simulink model "librarySample"  (R2017b)
settings: Solver=ode3  StartTime=0.0  StopTime=10.0  FixedStep=0.001  RelTol=1e-3
settings Model: Creator=Administrator  LastModifiedBy=Administrator

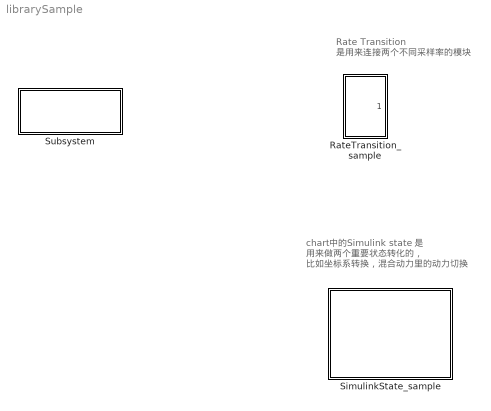
== system librarySample ==
  note: chart中的Simulink state 是
      | 用来做两个重要状态转化的，
      | 比如坐标系转换，混合动力里的动力切换
  note: Rate Transition
      | 是用来连接两个不同采样率的模块
  RateTransition_sample : Subsystem
  SimulinkState_sample : Subsystem
  Subsystem : Subsystem

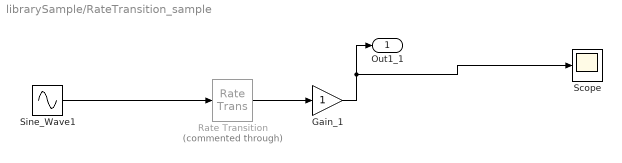
== system librarySample/RateTransition_sample ==
  Gain_1 : Gain
  Rate Transition : RateTransition  Commented=through
  Scope : Scope
  Sine_Wave1 : Sin  SampleTime=0.01
  Out1_1 : Outport  SampleTime=0.1
  wires:
  Sine_Wave1/1 -> Rate Transition/1
  Rate Transition/1 -> Gain_1/1
  Gain_1/1 -> Scope/1, Out1_1/1

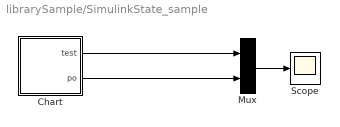
== system librarySample/SimulinkState_sample ==
  Chart : Stateflow chart  TreatAsAtomicUnit=on
  Mux : Mux  Inputs=2
  Scope : Scope
  wires:
  Chart/2(po) -> Mux/2
  Mux/1 -> Scope/1
  Chart/1(test) -> Mux/1

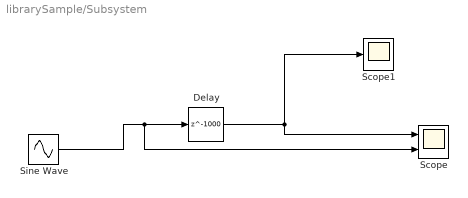
== system librarySample/Subsystem ==
  Delay : Delay  DelayLength=1000
  Scope : Scope  NumInputPorts=2
  Scope1 : Scope
  Sine Wave : Sin  SampleTime=0
  wires:
  Sine Wave/1 -> Scope/2, Delay/1
  Delay/1 -> Scope/1, Scope1/1

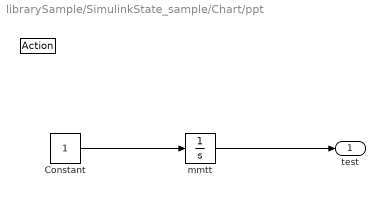
== system librarySample/SimulinkState_sample/Chart/ppt ==
  " " : ActionPort
      settings: CopyFcn=Stateflow.SLINSF.SimulinkMan.removeBlockPreDeleteFcn  PreDeleteFcn=Stateflow.SLINSF.SimulinkMan.unsafePredeleteFcn
  Constant : Constant
  mmtt : Integrator  ContinuousStateAttributes='m'
  test : Outport
  wires:
  Constant/1 -> mmtt/1
  mmtt/1 -> test/1

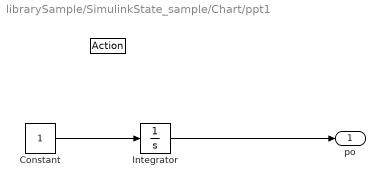
== system librarySample/SimulinkState_sample/Chart/ppt1 ==
  " " : ActionPort
      settings: CopyFcn=Stateflow.SLINSF.SimulinkMan.removeBlockPreDeleteFcn  PreDeleteFcn=Stateflow.SLINSF.SimulinkMan.unsafePredeleteFcn
  Constant : Constant
  Integrator : Integrator  ContinuousStateAttributes='tt'
  po : Outport
  wires:
  Integrator/1 -> po/1
  Constant/1 -> Integrator/1

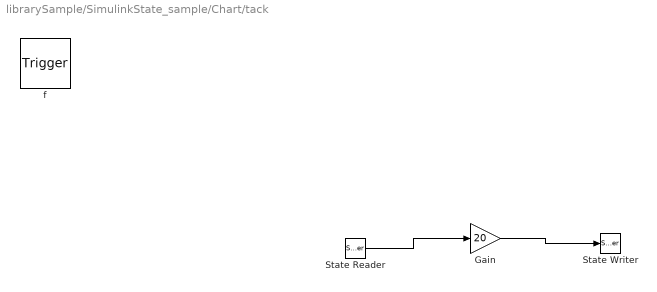
== system librarySample/SimulinkState_sample/Chart/tack ==
  f : TriggerPort  TriggerType=function-call  VariantControl=(inherit)
      settings: CopyFcn=Stateflow.SLINSF.SimulinkMan.removeBlockPreDeleteFcn  PreDeleteFcn=Stateflow.SLINSF.SimulinkMan.unsafePredeleteFcn
  Gain : Gain  Gain=20
  State Reader : StateReader  StateOwnerBlock=../../ppt/mmtt
  State Writer : StateWriter  StateOwnerBlock=../../ppt1/Integrator
  wires:
  State Reader/1 -> Gain/1
  Gain/1 -> State Writer/1

== stateflow chart librarySample/SimulinkState_sample/Chart ==
  state tack [function]
  state ppt
  state ppt1
  (default) -> ppt
  ppt -> ppt1 : [ppt.m(1)>2]{tack()}
  data: sf_internal_action_state_placeholder_data local double size=1 =0; m local; sf_internal_action_state_placeholder_data local double size=1 =0; test output; po output
